simulink model "Circulation_Model"  (Simulink 8.7)
settings: Solver=VariableStepAuto  SolverMode=SingleTasking  StartTime=0.0  StopTime=10.0  RelTol=1e-3
libraries: powerlib x71
settings Model: Creator=SHANY  LastModifiedBy=SHANY
settings DataIOCC: LimitDataPoints=off  SaveFormat=Dataset
settings DebuggingCC: UnderspecifiedInitializationDetection=Simplified  MergeDetectMultiDrivingBlocksExec=error  SFUnexpectedBacktrackingDiag=error  SFNoUnconditionalDefaultTransitionDiag=error
settings HardwareCC: ProdBitPerPointer=64  ProdLargestAtomicFloat=Float  ProdIntDivRoundTo=Zero  ProdEndianess=LittleEndian  ProdWordSize=64  ProdHWDeviceType=Intel->x86-64 (Windows64)
settings ModelReferenceCC: PropagateSignalLabelsOutOfModel=on
settings GRTTargetCC: TargetLangStandard=C99 (ISO)  GeneratePreprocessorConditionals=Use local settings
settings ConfigComp: CovMetricSettings=dwe  CovHtmlReporting=off  CovSaveCumulativeToWorkspaceVar=off  CovSaveSingleToWorkspaceVar=off  CovModelRefEnable=off  CovExternalEMLEnable=on

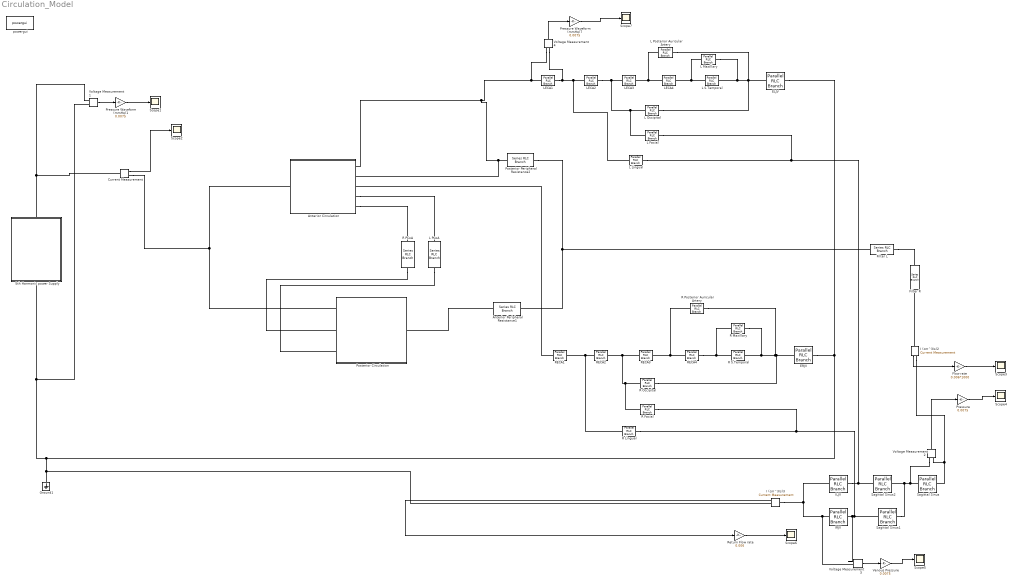
== system Circulation_Model ==
  5th Harmonic power Supply : Subsystem
  Anterior Circulation : Subsystem
  Anterior Peripheral Resistance1 : powerlib/Elements/Series RLC Branch  LConnTagsString=__new0  RConnTagsString=__new0  BranchType=R  Resistance=1  Inductance=1e-3  SetiL0=off  InitialCurrent=0  Capacitance=1e-6  Setx0=off  InitialVoltage=0  Measurements=None
  Current Measurement : powerlib/Measurements/Current Measurement  PhasorSimulation=off  OutputType=Complex  PSBequivalent=0
  ELJV : powerlib/Elements/Parallel RLC Branch  LConnTagsString=a  RConnTagsString=__new0  BranchType=R  Resistance=2500  Inductance=1e-3  SetiL0=off  InitialCurrent=0  Capacitance=1e-6  Setx0=off  InitialVoltage=0  Measurements=None
  ERJV : powerlib/Elements/Parallel RLC Branch  LConnTagsString=a  RConnTagsString=__new0  BranchType=R  Resistance=2500  Inductance=1e-3  SetiL0=off  InitialCurrent=0  Capacitance=1e-6  Setx0=off  InitialVoltage=0  Measurements=None
  Filter L : powerlib/Elements/Series RLC Branch  LConnTagsString=__new0  RConnTagsString=__new0  BranchType=L  Resistance=2e9  Inductance=100  SetiL0=off  InitialCurrent=6.69e-006  Capacitance=1e-6  Setx0=off  InitialVoltage=0  Measurements=None
  Filter R : powerlib/Elements/Series RLC Branch  LConnTagsString=__new0  RConnTagsString=__new0  BranchType=R  Resistance=550  Inductance=1e-3  SetiL0=off  InitialCurrent=0  Capacitance=0.00012803e-6  Setx0=off  InitialVoltage=13332.2368  Measurements=None
  Flow rate : Gain  Gain=0.006*1000
  Ground1 : powerlib/Elements/Ground  LConnTagsString=a
  I (cm^3/s)2 : powerlib/Measurements/Current Measurement  PhasorSimulation=off  OutputType=Complex  PSBequivalent=0
  I (cm^3/s)3 : powerlib/Measurements/Current Measurement  PhasorSimulation=off  OutputType=Complex  PSBequivalent=0
  ILJV : powerlib/Elements/Parallel RLC Branch  LConnTagsString=a  RConnTagsString=__new0  BranchType=R  Resistance=10  Inductance=1e-3  SetiL0=off  InitialCurrent=0  Capacitance=1e-6  Setx0=off  InitialVoltage=0  Measurements=None
  IRJV : powerlib/Elements/Parallel RLC Branch  LConnTagsString=a  RConnTagsString=__new0  BranchType=R  Resistance=10  Inductance=1e-3  SetiL0=off  InitialCurrent=0  Capacitance=1e-6  Setx0=off  InitialVoltage=0  Measurements=None
  L Facial : powerlib/Elements/Parallel RLC Branch  LConnTagsString=a  RConnTagsString=__new0  BranchType=R  Resistance=2000  Inductance=1e-3  SetiL0=off  InitialCurrent=0  Capacitance=200e-3  Setx0=off  InitialVoltage=0  Measurements=None
  L Lingual : powerlib/Elements/Parallel RLC Branch  LConnTagsString=a  RConnTagsString=__new0  BranchType=R  Resistance=2000  Inductance=1e-3  SetiL0=off  InitialCurrent=0  Capacitance=200e-3  Setx0=off  InitialVoltage=0  Measurements=None
  L Maxillary : powerlib/Elements/Parallel RLC Branch  LConnTagsString=a  RConnTagsString=__new0  BranchType=R  Resistance=1000  Inductance=1e-3  SetiL0=off  InitialCurrent=0  Capacitance=200e-3  Setx0=off  InitialVoltage=0  Measurements=None
  L Occipital : powerlib/Elements/Parallel RLC Branch  LConnTagsString=a  RConnTagsString=__new0  BranchType=R  Resistance=2000  Inductance=1e-3  SetiL0=off  InitialCurrent=0  Capacitance=200e-3  Setx0=off  InitialVoltage=0  Measurements=None
  "L PCoA " : powerlib/Elements/Series RLC Branch  LConnTagsString=__new0  RConnTagsString=__new0  BranchType=R  Resistance=1  Inductance=1e-3  SetiL0=off  InitialCurrent=0  Capacitance=1e-6  Setx0=off  InitialVoltage=0  Measurements=None
  L Posterior Auricular Artery : powerlib/Elements/Parallel RLC Branch  LConnTagsString=a  RConnTagsString=__new0  BranchType=R  Resistance=1000  Inductance=1e-3  SetiL0=off  InitialCurrent=0  Capacitance=200e-3  Setx0=off  InitialVoltage=0  Measurements=None
  L S.Temporal : powerlib/Elements/Parallel RLC Branch  LConnTagsString=a  RConnTagsString=__new0  BranchType=R  Resistance=1000  Inductance=1e-3  SetiL0=off  InitialCurrent=0  Capacitance=200e-3  Setx0=off  InitialVoltage=0  Measurements=None
  LECA1 : powerlib/Elements/Parallel RLC Branch  LConnTagsString=a  RConnTagsString=__new0  BranchType=R  Resistance=2500  Inductance=1e-3  SetiL0=off  InitialCurrent=0  Capacitance=200e-3  Setx0=off  InitialVoltage=0  Measurements=None
  LECA2 : powerlib/Elements/Parallel RLC Branch  LConnTagsString=a  RConnTagsString=__new0  BranchType=R  Resistance=1000  Inductance=1e-3  SetiL0=off  InitialCurrent=0  Capacitance=200e-3  Setx0=off  InitialVoltage=0  Measurements=None
  LECA3 : powerlib/Elements/Parallel RLC Branch  LConnTagsString=a  RConnTagsString=__new0  BranchType=R  Resistance=1000  Inductance=1e-3  SetiL0=off  InitialCurrent=0  Capacitance=200e-3  Setx0=off  InitialVoltage=0  Measurements=None
  LECA4 : powerlib/Elements/Parallel RLC Branch  LConnTagsString=a  RConnTagsString=__new0  BranchType=R  Resistance=1000  Inductance=1e-3  SetiL0=off  InitialCurrent=0  Capacitance=200e-3  Setx0=off  InitialVoltage=0  Measurements=None
  Posterior Circulation : Subsystem
  "Posterior Peripheral Resistance2 " : powerlib/Elements/Series RLC Branch  LConnTagsString=__new0  RConnTagsString=__new0  BranchType=R  Resistance=1  Inductance=1e-3  SetiL0=off  InitialCurrent=0  Capacitance=1e-6  Setx0=off  InitialVoltage=0  Measurements=None
  Pressure : Gain  Gain=0.0075
  Pressure Waveform (mmHg)1 : Gain  Gain=0.0075
  Pressure Waveform (mmHg)7 : Gain  Gain=0.0075
  R Facial : powerlib/Elements/Parallel RLC Branch  LConnTagsString=a  RConnTagsString=__new0  BranchType=R  Resistance=2000  Inductance=1e-3  SetiL0=off  InitialCurrent=0  Capacitance=200e-3  Setx0=off  InitialVoltage=0  Measurements=None
  R Lingual : powerlib/Elements/Parallel RLC Branch  LConnTagsString=a  RConnTagsString=__new0  BranchType=R  Resistance=2000  Inductance=1e-3  SetiL0=off  InitialCurrent=0  Capacitance=200e-3  Setx0=off  InitialVoltage=0  Measurements=None
  R Maxillary : powerlib/Elements/Parallel RLC Branch  LConnTagsString=a  RConnTagsString=__new0  BranchType=R  Resistance=1000  Inductance=1e-3  SetiL0=off  InitialCurrent=0  Capacitance=200e-3  Setx0=off  InitialVoltage=0  Measurements=None
  R Occipital : powerlib/Elements/Parallel RLC Branch  LConnTagsString=a  RConnTagsString=__new0  BranchType=R  Resistance=2000  Inductance=1e-3  SetiL0=off  InitialCurrent=0  Capacitance=200e-3  Setx0=off  InitialVoltage=0  Measurements=None
  R PCoA : powerlib/Elements/Series RLC Branch  LConnTagsString=__new0  RConnTagsString=__new0  BranchType=R  Resistance=1  Inductance=1e-3  SetiL0=off  InitialCurrent=0  Capacitance=1e-6  Setx0=off  InitialVoltage=0  Measurements=None
  R Posterior Auricular Artery : powerlib/Elements/Parallel RLC Branch  LConnTagsString=a  RConnTagsString=__new0  BranchType=R  Resistance=1000  Inductance=1e-3  SetiL0=off  InitialCurrent=0  Capacitance=200e-3  Setx0=off  InitialVoltage=0  Measurements=None
  R S.Temporal : powerlib/Elements/Parallel RLC Branch  LConnTagsString=a  RConnTagsString=__new0  BranchType=R  Resistance=1000  Inductance=1e-3  SetiL0=off  InitialCurrent=0  Capacitance=200e-3  Setx0=off  InitialVoltage=0  Measurements=None
  RECA1 : powerlib/Elements/Parallel RLC Branch  LConnTagsString=a  RConnTagsString=__new0  BranchType=R  Resistance=2500  Inductance=1e-3  SetiL0=off  InitialCurrent=0  Capacitance=200e-3  Setx0=off  InitialVoltage=0  Measurements=None
  RECA2 : powerlib/Elements/Parallel RLC Branch  LConnTagsString=a  RConnTagsString=__new0  BranchType=R  Resistance=1000  Inductance=1e-3  SetiL0=off  InitialCurrent=0  Capacitance=200e-3  Setx0=off  InitialVoltage=0  Measurements=None
  RECA3 : powerlib/Elements/Parallel RLC Branch  LConnTagsString=a  RConnTagsString=__new0  BranchType=R  Resistance=1000  Inductance=1e-3  SetiL0=off  InitialCurrent=0  Capacitance=200e-3  Setx0=off  InitialVoltage=0  Measurements=None
  RECA4 : powerlib/Elements/Parallel RLC Branch  LConnTagsString=a  RConnTagsString=__new0  BranchType=R  Resistance=1000  Inductance=1e-3  SetiL0=off  InitialCurrent=0  Capacitance=200e-3  Setx0=off  InitialVoltage=0  Measurements=None
  Return Flow rate : Gain  Gain=0.006
  Sagittal Sinus : powerlib/Elements/Parallel RLC Branch  LConnTagsString=a  RConnTagsString=__new0  BranchType=R  Resistance=50  Inductance=1e-3  SetiL0=off  InitialCurrent=0  Capacitance=1e-6  Setx0=off  InitialVoltage=0  Measurements=None
  Sagittal Sinus1 : powerlib/Elements/Parallel RLC Branch  LConnTagsString=a  RConnTagsString=__new0  BranchType=R  Resistance=50  Inductance=1e-3  SetiL0=off  InitialCurrent=0  Capacitance=1e-6  Setx0=off  InitialVoltage=0  Measurements=None
  Sagittal Sinus2 : powerlib/Elements/Parallel RLC Branch  LConnTagsString=a  RConnTagsString=__new0  BranchType=R  Resistance=50  Inductance=1e-3  SetiL0=off  InitialCurrent=0  Capacitance=1e-6  Setx0=off  InitialVoltage=0  Measurements=None
  Scope{1..7} (7 alike) : Scope
  Venous Pressure : Gain  Gain=0.0075
  Voltage Measurement{1..4} (4 alike) : powerlib/Measurements/Voltage Measurement  PhasorSimulation=off  OutputType=Complex  PSBequivalent=0
  powergui : powerlib/powergui  Priority=1  SimulationMode=Continuous  SampleTime=50e-6  frequency=60  Iterations=50  frequencyindice=1  Pbase=100e6  ErrMax=1e-4  UnitsV=kV  UnitsW=MW  buscounter=0  FunctionMessages=off  echomessages=off  EnableUseOfTLC=off  CurrentSourceSwitches=off  DisableSnubberDevices=off  DisableRonSwitches=off  DisableVfSwitches=off  DisplayEquations=off  SolverType=Tustin/Backward Euler (TBE)  Interpol=off  ExternalGateDelay=off  methode=off  Ts=100  x0status=blocks  SPID=on  SwTol=0  HookPort=off  RestoreLinks=warning  ResistiveCurrentMeasurement=off  Frange=[0:2:500]  Ylog=off  Xlog=on  ShowGrid=off  save=off  variable=ZData  structure=0  ZoomFFT=off  StartTime=0.0  cycles=1  DisplayStyle=1  fundamental=60  FreqAxis=off  MaxFrequency=1000  frequencyindicesteady=1  RmsSteady=1  display=off
  wires:
  Voltage Measurement1/1 -> Pressure Waveform (mmHg)1/1
  Pressure Waveform (mmHg)1/1 -> Scope1/1
  Current Measurement/1 -> Scope2/1
  I (cm^3/s)2/1 -> Flow rate/1
  Flow rate/1 -> Scope3/1
  Voltage Measurement2/1 -> Pressure/1
  Pressure/1 -> Scope4/1
  Voltage Measurement3/1 -> Venous Pressure/1
  Venous Pressure/1 -> Scope5/1
  Return Flow rate/1 -> Scope6/1
  I (cm^3/s)3/1 -> Return Flow rate/1
  Voltage Measurement4/1 -> Pressure Waveform (mmHg)7/1
  Pressure Waveform (mmHg)7/1 -> Scope7/1
  connections:
  Current Measurement/RConn1 -- Anterior Circulation/LConn1 -- Posterior Circulation/LConn1
  "Posterior Peripheral Resistance2 "/RConn1 -- Anterior Peripheral Resistance1/RConn1 -- Filter L/LConn1
  L S.Temporal/LConn1 -- L Maxillary/LConn1 -- LECA4/RConn1
  ELJV/RConn1 -- L Occipital/RConn1 -- L Posterior Auricular Artery/RConn1 -- L Maxillary/RConn1 -- L S.Temporal/RConn1
  LECA4/LConn1 -- L Posterior Auricular Artery/LConn1 -- LECA3/RConn1
  LECA2/RConn1 -- L Facial/LConn1 -- L Occipital/LConn1 -- LECA3/LConn1
  LECA1/RConn1 -- Voltage Measurement4/LConn2 -- L Lingual/LConn1 -- LECA2/LConn1
  RECA4/RConn1 -- R Maxillary/LConn1 -- R S.Temporal/LConn1
  ERJV/RConn1 -- R Occipital/RConn1 -- R Posterior Auricular Artery/RConn1 -- R Maxillary/RConn1 -- R S.Temporal/RConn1
  RECA4/LConn1 -- R Posterior Auricular Artery/LConn1 -- RECA3/RConn1
  RECA3/LConn1 -- R Facial/LConn1 -- R Occipital/LConn1 -- RECA2/RConn1
  RECA2/LConn1 -- R Lingual/LConn1 -- RECA1/RConn1
  "Posterior Peripheral Resistance2 "/LConn1 -- Voltage Measurement4/LConn1 -- LECA1/LConn1 -- Anterior Circulation/RConn1 -- Anterior Circulation/RConn2
  R PCoA/RConn1 -- Posterior Circulation/LConn2
  "L PCoA "/RConn1 -- Posterior Circulation/LConn3
  Anterior Peripheral Resistance1/LConn1 -- Posterior Circulation/RConn1
  5th Harmonic power Supply/RConn1 -- Current Measurement/LConn1 -- Voltage Measurement1/LConn1
  ILJV/LConn1 -- L Facial/RConn1 -- L Lingual/RConn1 -- Sagittal Sinus2/RConn1
  IRJV/LConn1 -- Voltage Measurement3/LConn1 -- Sagittal Sinus1/RConn1 -- R Facial/RConn1 -- R Lingual/RConn1
  Filter L/RConn1 -- Filter R/RConn1
  RECA1/LConn1 -- Anterior Circulation/RConn3
  Anterior Circulation/RConn4 -- "L PCoA "/LConn1
  Anterior Circulation/RConn5 -- R PCoA/LConn1
  I (cm^3/s)2/LConn1 -- Filter R/LConn1
  I (cm^3/s)2/RConn1 -- Voltage Measurement2/LConn2 -- Sagittal Sinus/LConn1
  Sagittal Sinus/RConn1 -- Voltage Measurement2/LConn1 -- Sagittal Sinus1/LConn1 -- Sagittal Sinus2/LConn1
  ILJV/RConn1 -- I (cm^3/s)3/LConn1 -- Voltage Measurement3/LConn2 -- IRJV/RConn1
  ELJV/LConn1 -- ERJV/LConn1 -- Voltage Measurement1/LConn2 -- 5th Harmonic power Supply/LConn1 -- I (cm^3/s)3/RConn1 -- Ground1/LConn1

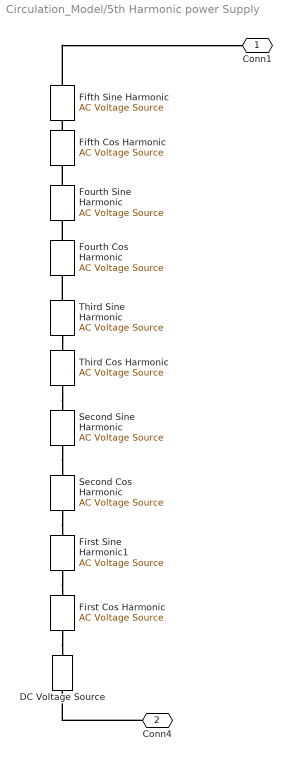
== system Circulation_Model/5th Harmonic power Supply ==
  DC Voltage Source : powerlib/Electrical Sources/DC Voltage Source  Amplitude=13128  Measurements=None
  Fifth Cos Harmonic : powerlib/Electrical Sources/AC Voltage Source  Amplitude=68  Phase=90  Frequency=5  SampleTime=0  Measurements=None  BusType=swing  Pref=10e3  Qref=0  Qmin=-inf  Qmax=+inf
  Fifth Sine Harmonic : powerlib/Electrical Sources/AC Voltage Source  Amplitude=-50.6  Phase=0  Frequency=5  SampleTime=0  Measurements=None  BusType=swing  Pref=10e3  Qref=0  Qmin=-inf  Qmax=+inf
  First Cos Harmonic : powerlib/Electrical Sources/AC Voltage Source  Amplitude=-423  Phase=90  Frequency=1  SampleTime=0  Measurements=None  BusType=swing  Pref=10e3  Qref=0  Qmin=-inf  Qmax=+inf
  First Sine Harmonic1 : powerlib/Electrical Sources/AC Voltage Source  Amplitude=1417  Phase=0  Frequency=1  SampleTime=0  Measurements=None  BusType=swing  Pref=10e3  Qref=0  Qmin=-inf  Qmax=+inf
  Fourth Cos Harmonic : powerlib/Electrical Sources/AC Voltage Source  Amplitude=-326  Phase=90  Frequency=4  SampleTime=0  Measurements=None  BusType=swing  Pref=10e3  Qref=0  Qmin=-inf  Qmax=+inf
  Fourth Sine Harmonic : powerlib/Electrical Sources/AC Voltage Source  Amplitude=-238  Phase=0  Frequency=4  SampleTime=0  Measurements=None  BusType=swing  Pref=10e3  Qref=0  Qmin=-inf  Qmax=+inf
  Second Cos Harmonic : powerlib/Electrical Sources/AC Voltage Source  Amplitude=-418  Phase=90  Frequency=2  SampleTime=0  Measurements=None  BusType=swing  Pref=10e3  Qref=0  Qmin=-inf  Qmax=+inf
  Second Sine Harmonic : powerlib/Electrical Sources/AC Voltage Source  Amplitude=747  Phase=0  Frequency=2  SampleTime=0  Measurements=None  BusType=swing  Pref=10e3  Qref=0  Qmin=-inf  Qmax=+inf
  Third Cos Harmonic : powerlib/Electrical Sources/AC Voltage Source  Amplitude=-615  Phase=90  Frequency=3  SampleTime=0  Measurements=None  BusType=swing  Pref=10e3  Qref=0  Qmin=-inf  Qmax=+inf
  "Third Sine Harmonic " : powerlib/Electrical Sources/AC Voltage Source  Amplitude=312  Phase=0  Frequency=3  SampleTime=0  Measurements=None  BusType=swing  Pref=10e3  Qref=0  Qmin=-inf  Qmax=+inf
  Conn1 : PMIOPort  Side=Right
  Conn4 : PMIOPort  Port=2  Side=Left
  connections:
  Third Cos Harmonic/LConn1 -- Second Sine Harmonic/RConn1
  "Third Sine Harmonic "/LConn1 -- Third Cos Harmonic/RConn1
  First Sine Harmonic1/LConn1 -- First Cos Harmonic/RConn1
  Fourth Cos Harmonic/RConn1 -- Fourth Sine Harmonic/LConn1
  "Third Sine Harmonic "/RConn1 -- Fourth Cos Harmonic/LConn1
  Second Cos Harmonic/LConn1 -- First Sine Harmonic1/RConn1
  Second Sine Harmonic/LConn1 -- Second Cos Harmonic/RConn1
  First Cos Harmonic/LConn1 -- DC Voltage Source/RConn1
  Fourth Sine Harmonic/RConn1 -- Fifth Cos Harmonic/LConn1
  Conn4/RConn1 -- DC Voltage Source/LConn1
  Fifth Cos Harmonic/RConn1 -- Conn1/RConn1

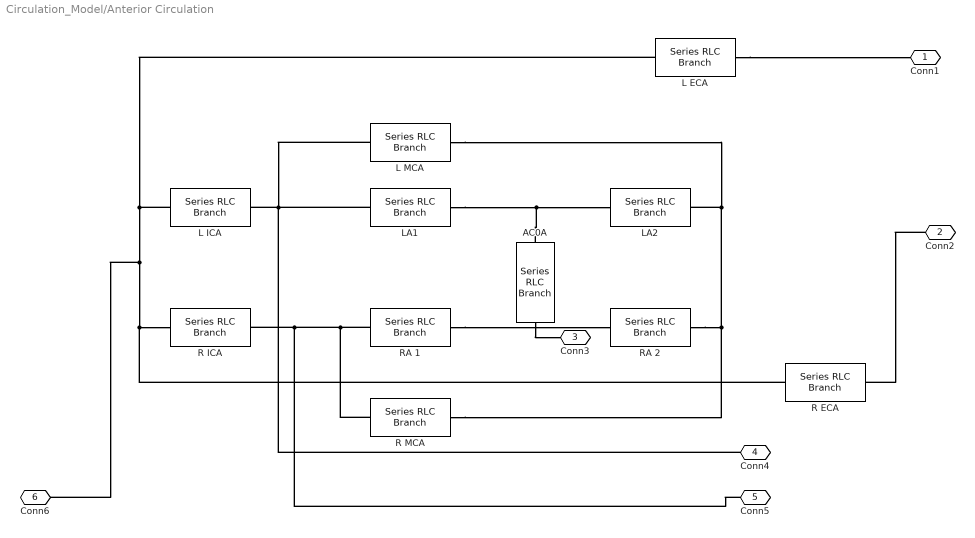
== system Circulation_Model/Anterior Circulation ==
  AC0A : powerlib/Elements/Series RLC Branch  LConnTagsString=__new0  RConnTagsString=__new0  BranchType=R  Resistance=2000  Inductance=1e-3  SetiL0=off  InitialCurrent=0  Capacitance=1e-6  Setx0=off  InitialVoltage=0  Measurements=Branch voltage and current
  L ECA : powerlib/Elements/Series RLC Branch  LConnTagsString=__new0  RConnTagsString=__new0  BranchType=R  Resistance=2000  Inductance=1e-3  SetiL0=off  InitialCurrent=0  Capacitance=1e-6  Setx0=off  InitialVoltage=0  Measurements=Branch voltage and current
  "L ICA " : powerlib/Elements/Series RLC Branch  LConnTagsString=__new0  RConnTagsString=__new0  BranchType=R  Resistance=10  Inductance=1e-3  SetiL0=off  InitialCurrent=0  Capacitance=1e-6  Setx0=off  InitialVoltage=0  Measurements=None
  L MCA : powerlib/Elements/Series RLC Branch  LConnTagsString=__new0  RConnTagsString=__new0  BranchType=R  Resistance=400  Inductance=1e-3  SetiL0=off  InitialCurrent=0  Capacitance=1e-6  Setx0=off  InitialVoltage=0  Measurements=Branch voltage and current
  "LA1 " : powerlib/Elements/Series RLC Branch  LConnTagsString=__new0  RConnTagsString=__new0  BranchType=R  Resistance=250  Inductance=1e-3  SetiL0=off  InitialCurrent=0  Capacitance=1e-6  Setx0=off  InitialVoltage=0  Measurements=Branch voltage and current
  LA2 : powerlib/Elements/Series RLC Branch  LConnTagsString=__new0  RConnTagsString=__new0  BranchType=R  Resistance=300  Inductance=1e-3  SetiL0=off  InitialCurrent=0  Capacitance=1e-6  Setx0=off  InitialVoltage=0  Measurements=Branch voltage and current
  R ECA : powerlib/Elements/Series RLC Branch  LConnTagsString=__new0  RConnTagsString=__new0  BranchType=R  Resistance=2000  Inductance=1e-3  SetiL0=off  InitialCurrent=0  Capacitance=1e-6  Setx0=off  InitialVoltage=0  Measurements=Branch voltage and current
  R ICA : powerlib/Elements/Series RLC Branch  LConnTagsString=__new0  RConnTagsString=__new0  BranchType=R  Resistance=10  Inductance=1e-3  SetiL0=off  InitialCurrent=0  Capacitance=1e-6  Setx0=off  InitialVoltage=0  Measurements=Branch voltage and current
  R MCA : powerlib/Elements/Series RLC Branch  LConnTagsString=__new0  RConnTagsString=__new0  BranchType=R  Resistance=400  Inductance=1e-3  SetiL0=off  InitialCurrent=0  Capacitance=1e-6  Setx0=off  InitialVoltage=0  Measurements=Branch voltage and current
  RA 1 : powerlib/Elements/Series RLC Branch  LConnTagsString=__new0  RConnTagsString=__new0  BranchType=R  Resistance=250  Inductance=1e-3  SetiL0=off  InitialCurrent=0  Capacitance=1e-6  Setx0=off  InitialVoltage=0  Measurements=Branch voltage and current
  "RA 2 " : powerlib/Elements/Series RLC Branch  LConnTagsString=__new0  RConnTagsString=__new0  BranchType=R  Resistance=300  Inductance=1e-3  SetiL0=off  InitialCurrent=0  Capacitance=1e-6  Setx0=off  InitialVoltage=0  Measurements=Branch voltage and current
  Conn1 : PMIOPort  Side=Right
  Conn2 : PMIOPort  Port=2  Side=Right
  Conn3 : PMIOPort  Port=3  Side=Right
  Conn4 : PMIOPort  Port=4  Side=Right
  Conn5 : PMIOPort  Port=5  Side=Right
  Conn6 : PMIOPort  Port=6  Side=Left
  connections:
  Conn2/RConn1 -- R ECA/RConn1
  RA 1/LConn1 -- R MCA/LConn1 -- Conn5/RConn1 -- R ICA/RConn1
  "LA1 "/RConn1 -- AC0A/LConn1 -- LA2/LConn1
  L MCA/LConn1 -- Conn4/RConn1 -- "L ICA "/RConn1 -- "LA1 "/LConn1
  RA 1/RConn1 -- "RA 2 "/LConn1
  "RA 2 "/RConn1 -- R MCA/RConn1 -- L MCA/RConn1 -- LA2/RConn1
  AC0A/RConn1 -- Conn3/RConn1
  R ECA/LConn1 -- Conn6/RConn1 -- L ECA/LConn1 -- "L ICA "/LConn1 -- R ICA/LConn1
  L ECA/RConn1 -- Conn1/RConn1

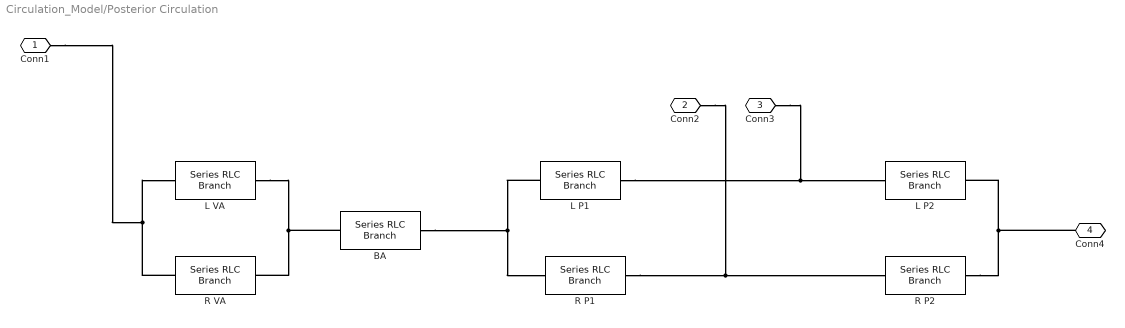
== system Circulation_Model/Posterior Circulation ==
  BA : powerlib/Elements/Series RLC Branch  LConnTagsString=__new0  RConnTagsString=__new0  BranchType=R  Resistance=1  Inductance=1e-3  SetiL0=off  InitialCurrent=0  Capacitance=1e-6  Setx0=off  InitialVoltage=0  Measurements=None
  L P1 : powerlib/Elements/Series RLC Branch  LConnTagsString=__new0  RConnTagsString=__new0  BranchType=R  Resistance=1  Inductance=1e-3  SetiL0=off  InitialCurrent=0  Capacitance=1e-6  Setx0=off  InitialVoltage=0  Measurements=None
  L P2 : powerlib/Elements/Series RLC Branch  LConnTagsString=__new0  RConnTagsString=__new0  BranchType=R  Resistance=1  Inductance=1e-3  SetiL0=off  InitialCurrent=0  Capacitance=1e-6  Setx0=off  InitialVoltage=0  Measurements=None
  "L VA " : powerlib/Elements/Series RLC Branch  LConnTagsString=__new0  RConnTagsString=__new0  BranchType=R  Resistance=1  Inductance=1e-3  SetiL0=off  InitialCurrent=0  Capacitance=1e-6  Setx0=off  InitialVoltage=0  Measurements=Branch voltage and current
  R P1 : powerlib/Elements/Series RLC Branch  LConnTagsString=__new0  RConnTagsString=__new0  BranchType=R  Resistance=1  Inductance=1e-3  SetiL0=off  InitialCurrent=0  Capacitance=1e-6  Setx0=off  InitialVoltage=0  Measurements=None
  R P2 : powerlib/Elements/Series RLC Branch  LConnTagsString=__new0  RConnTagsString=__new0  BranchType=R  Resistance=1  Inductance=1e-3  SetiL0=off  InitialCurrent=0  Capacitance=1e-6  Setx0=off  InitialVoltage=0  Measurements=None
  "R VA " : powerlib/Elements/Series RLC Branch  LConnTagsString=__new0  RConnTagsString=__new0  BranchType=R  Resistance=1  Inductance=1e-3  SetiL0=off  InitialCurrent=0  Capacitance=1e-6  Setx0=off  InitialVoltage=0  Measurements=None
  Conn1 : PMIOPort  Side=Left
  Conn2 : PMIOPort  Port=2  Side=Left
  Conn3 : PMIOPort  Port=3  Side=Left
  Conn4 : PMIOPort  Port=4  Side=Right
  connections:
  "R VA "/LConn1 -- Conn1/RConn1 -- "L VA "/LConn1
  L P1/RConn1 -- Conn3/RConn1 -- L P2/LConn1
  R P2/RConn1 -- Conn4/RConn1 -- L P2/RConn1
  "L VA "/RConn1 -- BA/LConn1 -- "R VA "/RConn1
  R P1/RConn1 -- Conn2/RConn1 -- R P2/LConn1
  L P1/LConn1 -- BA/RConn1 -- R P1/LConn1
